simulink model "two_parallel_half_model_simscape"  (R2023b)
settings: Solver=ode1be  StartTime=0.0  StopTime=simlength  FixedStep=ts_sim  MaxStep=ts_sim
values from neighbouring files (symbols this model uses):
  fPWM_INV = 10e3    (= 10000)    [init_model.m]
  I_FS = Iout_ac_rms_nom * sqrt(2) * margin_factor    [init_model.m]
  ki_i_inv = 18    [init_model.m]
  ki_v_inv = 12.5    [init_model.m]
  kp_i_inv = 0.1    [init_model.m]
  kp_v_inv = 0.1    [init_model.m]
  LFu_ac = 125e-6*2    (= 0.00025)    [init_model.m]
  omega_grid = frequency_grid*2*pi    (= 314.159265359)    [init_model.m]
  RLFu_ac = 2e-3    (= 0.002)    [init_model.m]
  tc = ts_inv/200    (= 5e-07)    [init_model.m]
  ts_afe = ts_inv    (= 0.0001)    [init_model.m]
  ts_inv = tPWM_INV    (= 0.0001)    [init_model.m]
  ts_zvs = tPWM_ZVS*2    (= 0.0001)    [init_model.m]
  V_FS = Vout_dc_nom * margin_factor    (= 943)    [init_model.m]
  Vout_dc_nom = 820    [init_model.m]
undefined symbols (not defined in the file or in its folder): magnitude
libraries: fl_lib x43, nesl_utility x17
(part 1 of 2)
settings Model: SimulationMode=accelerator  Creator=LTNBDA  LastModifiedBy=dbagn
settings SolverCC: ZeroCrossControl=EnableAll  ZeroCrossAlgorithm=Adaptive  AlgebraicLoopSolver=TrustRegion  SolverResetMethod=Robust  AutoInsertRateTranBlk=on
settings DataIOCC: LimitDataPoints=on  MaxDataPoints=1  SaveFormat=Array  SignalLoggingSaveFormat=ModelDataLogs  SaveOutput=off  SignalLogging=off  DSMLogging=off  SaveTime=off  ReturnWorkspaceOutputs=off
settings OptimizationCC: ExpressionDepthLimit=2147483647  InitFltsAndDblsToZero=on  EfficientMapNaN2IntZero=off  LifeSpan=inf
settings DebuggingCC: SaveWithParameterizedLinksMsg=none  UnderspecifiedInitializationDetection=Classic  MergeDetectMultiDrivingBlocksExec=none  SignalResolutionControl=TryResolveAllWithWarning  SolverPrmCheckMsg=warning  MultiTaskDSMMsg=warning  MultiTaskCondExecSysMsg=none  MultiTaskRateTransMsg=warning  FcnCallInpInsideContextMsg=warning  StateNameClashWarn=warning  SFUnexpectedBacktrackingDiag=warning  SFNoUnconditionalDefaultTransitionDiag=warning  ArithmeticOperatorsInVariantConditions=warning
settings HardwareCC: ProdBitPerLong=64  ProdLargestAtomicFloat=None  ProdIntDivRoundTo=Undefined  ProdEndianess=Unspecified  ProdHWDeviceType=Generic->64-bit Embedded Processor (LP64)  TargetBitPerPointer=64  TargetBitPerSizeT=64  TargetBitPerPtrDiffT=64  TargetLongLongMode=on  TargetIntDivRoundTo=Zero  TargetEndianess=LittleEndian  TargetWordSize=64  TargetHWDeviceType=MATLAB Host  ProdEqTarget=off
settings ModelReferenceCC: EnableRefExpFcnMdlSchedulingChecks=on  PropagateSignalLabelsOutOfModel=off
settings SFSimCC: SimUseLocalCustomCode=off  CustomCodeUndefinedFunction=UseInterfaceOnly
settings RTWCC: RTWUseLocalCustomCode=off
settings CodeAppCC: MaxIdLength=128  StateflowObjectComments=on
settings GRTTargetCC: TargetLangStandard=C89/C90 (ANSI)  CombineOutputUpdateFcns=off  GRTInterface=on
settings ConfigComp: CovMetricSettings=dw  CovSaveCumulativeToWorkspaceVar=on  CovSaveSingleToWorkspaceVar=on  CovExternalEMLEnable=off
settings SimscapeCC: SimscapeNormalizeSystem=off

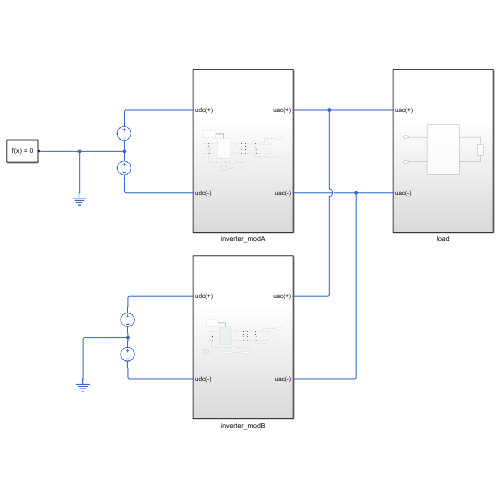
[thumbnail: Simulink's stored preview of the top-level diagram]
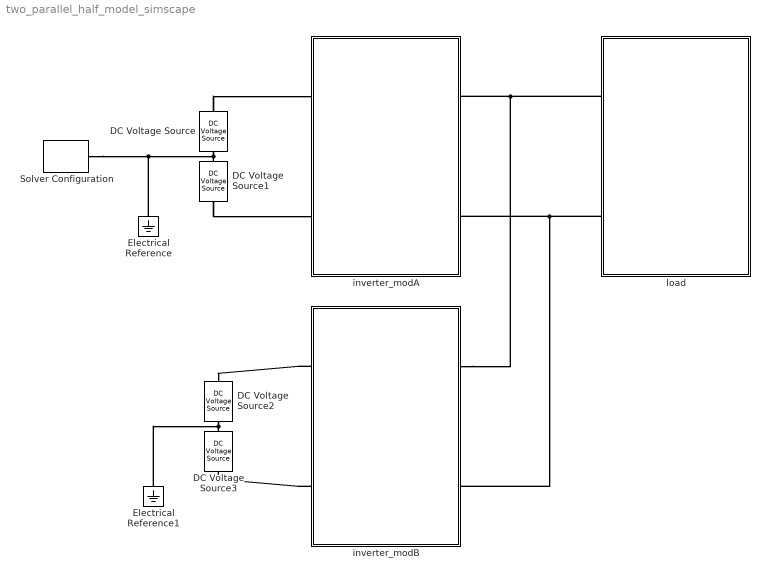
== system two_parallel_half_model_simscape ==
  DC Voltage Source{,1..3} (4 alike) : fl_lib/Electrical/Electrical Sources/DC Voltage Source  v0=Vout_dc_nom/2 V
  Electrical Reference : fl_lib/Electrical/Electrical Elements/Electrical Reference
  Electrical Reference1 : fl_lib/Electrical/Electrical Elements/Electrical Reference
  Solver Configuration : nesl_utility/Solver Configuration  PhysicalDomain=network_engine_domain  SubClassName=solver  LeftPortType=input  RightPortType=generic  Tones=[]  Harmonics=[]  SimulateNoise=off  Profile=off  UseLocalSampling=off  EnableSwitchedLinearOptims=on  FrequencyDomain=off  UseCCode=off  RelTol=0.001  AbsTol=0.001  MinStep=1e-09  ToWorkspace=off  RevertToSquareIcSolve=off  NumHomotopyIterations=100  PhasorMode=off  PhasorModeNumHarmonics=1  ConsistencySolver=NEWTON_FTOL  IndexReductionMethod=DerivativeReplacement  DoDC=on  ResidualTolerance=1e-09  ConsistencyTolSource=GLOBAL  ConsistencyAbsTol=0.001  ConsistencyRelTol=0.001  ConsistencyTolFactor=0.001  UseLocalSolver=on  LocalSolverChoice=NE_BACKWARD_EULER_ADVANCER  ResolveIndetEquations=on  FunctionEvalNumThread=1  LocalSolverSampleTime=ts_sim  DoFixedCost=on  MaxNonlinIter=3  MaxModeIter=2  ComputeImpulses=off  ImpulseIterations=2  LinearAlgebra=auto  LinearAlgebraNumThread=0  EquationFormulation=NE_TIME_EF  DelaysMemoryBudget=1024  AutomaticFiltering=on  FilteringTimeConstant=0.001  PartitionStorageMethod=AS_NEEDED  PartitionMemoryBudget=1024  PartitionMethod=ROBUST  MultibodyUseLocalSolver=off  MultibodyLocalSolverChoice=ODE1  MultibodyLocalSolverSampleTime=0.001
  inverter_modA : Subsystem
  inverter_modB : Subsystem
  load : Subsystem
  connections:
  DC Voltage Source/LConn1 -- inverter_modA/LConn1
  DC Voltage Source1/RConn1 -- inverter_modA/LConn2
  load/LConn1 -- inverter_modB/RConn1 -- inverter_modA/RConn1
  load/LConn2 -- inverter_modB/RConn2 -- inverter_modA/RConn2
  Solver Configuration/RConn1 -- Electrical Reference/LConn1 -- DC Voltage Source1/LConn1 -- DC Voltage Source/RConn1
  Electrical Reference1/LConn1 -- DC Voltage Source2/RConn1 -- DC Voltage Source3/LConn1
  inverter_modB/LConn2 -- DC Voltage Source3/RConn1
  inverter_modB/LConn1 -- DC Voltage Source2/LConn1

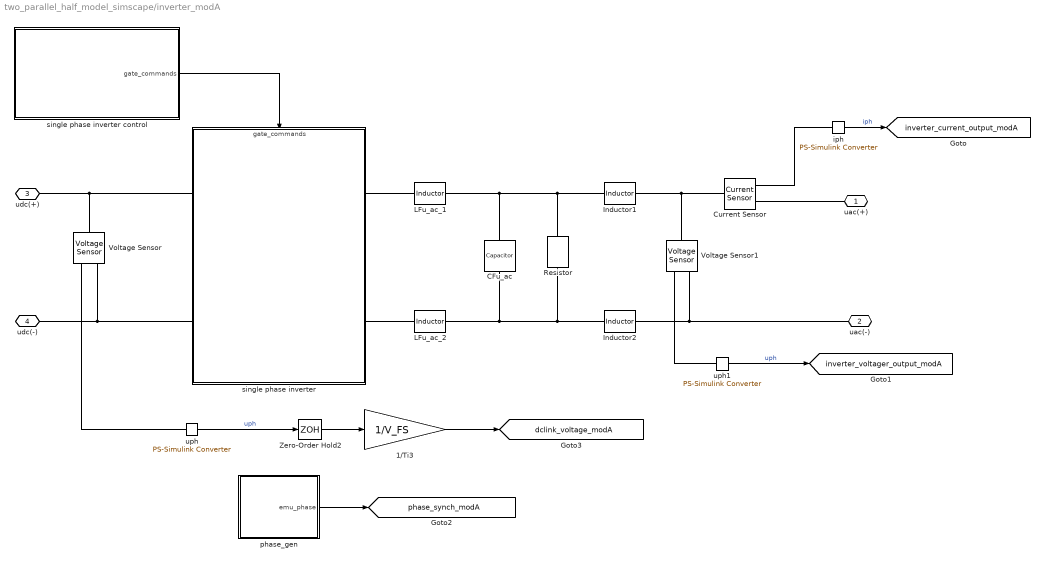
== system two_parallel_half_model_simscape/inverter_modA ==
  1/Ti3 : Gain  Gain=1/V_FS  SaturateOnIntegerOverflow=on  OutDataTypeStr=Inherit: Same as input  ParamDataTypeStr=Inherit: Same as input
  CFu_ac : fl_lib/Electrical/Electrical Elements/Capacitor  c=CFu_ac F  r=RCFu_ac Ohm  g=0 1/Ohm  i_specify=off  i_priority=None  i=0 A  i_nominal_specify=off  i_nominal_unit=A  i_nominal_value=1  v_specify=off  v_priority=None  v=0 V  v_nominal_specify=off  v_nominal_unit=V  v_nominal_value=1  vc_specify=off  vc_priority=High  vc=0 V  vc_nominal_specify=off  vc_nominal_unit=V  vc_nominal_value=1
  Current Sensor : fl_lib/Electrical/Electrical Sensors/Current Sensor
  Inductor1 : fl_lib/Electrical/Electrical Elements/Inductor  l=Lp H  r=0 Ohm  g=1e-9 1/Ohm  i_specify=off  i_priority=None  i=0 A  i_nominal_specify=off  i_nominal_unit=A  i_nominal_value=1  v_specify=off  v_priority=None  v=0 V  v_nominal_specify=off  v_nominal_unit=V  v_nominal_value=1  i_L_specify=off  i_L_priority=High  i_L=0 A  i_L_nominal_specify=off  i_L_nominal_unit=A  i_L_nominal_value=1
  Inductor2 : fl_lib/Electrical/Electrical Elements/Inductor  l=Lp H  r=0 Ohm  g=1e-9 1/Ohm  i_specify=off  i_priority=None  i=0 A  i_nominal_specify=off  i_nominal_unit=A  i_nominal_value=1  v_specify=off  v_priority=None  v=0 V  v_nominal_specify=off  v_nominal_unit=V  v_nominal_value=1  i_L_specify=off  i_L_priority=High  i_L=0 A  i_L_nominal_specify=off  i_L_nominal_unit=A  i_L_nominal_value=1
  LFu_ac_1 : fl_lib/Electrical/Electrical Elements/Inductor  l=LFu_ac/2 H  r=RLFu_ac/2 Ohm  g=0 1/Ohm  i_specify=off  i_priority=None  i=0 A  i_nominal_specify=off  i_nominal_unit=A  i_nominal_value=1  v_specify=off  v_priority=None  v=0 V  v_nominal_specify=off  v_nominal_unit=V  v_nominal_value=1  i_L_specify=off  i_L_priority=High  i_L=0 A  i_L_nominal_specify=off  i_L_nominal_unit=A  i_L_nominal_value=1
  LFu_ac_2 : fl_lib/Electrical/Electrical Elements/Inductor  l=LFu_ac/2 H  r=RLFu_ac/2 Ohm  g=0 1/Ohm  i_specify=off  i_priority=None  i=0 A  i_nominal_specify=off  i_nominal_unit=A  i_nominal_value=1  v_specify=off  v_priority=None  v=0 V  v_nominal_specify=off  v_nominal_unit=V  v_nominal_value=1  i_L_specify=off  i_L_priority=High  i_L=0 A  i_L_nominal_specify=off  i_L_nominal_unit=A  i_L_nominal_value=1
  Resistor : fl_lib/Electrical/Electrical Elements/Resistor  R=10e3 Ohm  i_specify=off  i_priority=None  i=0 A  i_nominal_specify=off  i_nominal_unit=A  i_nominal_value=1  v_specify=off  v_priority=None  v=0 V  v_nominal_specify=off  v_nominal_unit=V  v_nominal_value=1
  Voltage Sensor : fl_lib/Electrical/Electrical Sensors/Voltage Sensor
  Voltage Sensor1 : fl_lib/Electrical/Electrical Sensors/Voltage Sensor
  Zero-Order Hold2 : ZeroOrderHold  SampleTime=ts_zvs
  iph : nesl_utility/PS-Simulink Converter  PhysicalDomain=network_engine_domain  SubClassName=ps_output  LeftPortType=input  RightPortType=output  PseudoPeriodic=off  Frequencies=[]  VectorFormat=1-D array  Unit=A  AffineConversion=off
  phase_gen : Subsystem
  single phase inverter : Subsystem
      settings: PortSchema="{\"entries\":[{\"content\":{\"sides\":[{\"content\":{\"connectorIds\":[\"LConn1\",\"LConn2\"]},\"type\":\"ConnectorPlacement.EquallySpacedRectSide\",\"uuid\":\"4fcf4fea-d38f-431b-8a91-be3ce9782faf\"},{\"content\":{\"connectorIds\":[\"RConn1\",\"RConn2\"],\"side\":\"RIGHT\"},\"type\":\"ConnectorPlacement.EquallySpacedRectSide\",\"uuid\":\"0aa56277-92e9-4e3b-84c7-43398254a4d8\"},{\"content\":{\"connectorIds\":[\"In1\"],\"side\":\"TOP\"},\"type\":\"ConnectorPlacement.EquallySpacedRectSide\",\"uuid\":\"5cd150dc-bcaf-4cd7-b2a8-3db203726730\"}]},\"type\":\"ConnectorPlacement.EquallySpacedConnector\",\"uuid\":\"bf8194c4-c327-4d40-bea4-f1e7617f80b4\"}],\"packageUris\":[\"http://schema.mathworks.com/mf0/Connector/R2020b\"],\"version\":\"1.0\"}"
  single phase inverter control : Subsystem
  uph : nesl_utility/PS-Simulink Converter  PhysicalDomain=network_engine_domain  SubClassName=ps_output  LeftPortType=input  RightPortType=output  PseudoPeriodic=off  Frequencies=[]  VectorFormat=1-D array  Unit=V  AffineConversion=off
  uph1 : nesl_utility/PS-Simulink Converter  PhysicalDomain=network_engine_domain  SubClassName=ps_output  LeftPortType=input  RightPortType=output  PseudoPeriodic=off  Frequencies=[]  VectorFormat=1-D array  Unit=V  AffineConversion=off
  uac(+) : PMIOPort  Side=Right
  uac(-) : PMIOPort  Port=2  Side=Right
  udc(+) : PMIOPort  Port=3  Side=Left
  udc(-) : PMIOPort  Port=4  Side=Left
  tag scope: dclink_voltage_modA=global, inverter_current_output_modA=global, inverter_voltager_output_modA=global, phase_synch_modA=global
  wires:
  Zero-Order Hold2/1 -> 1/Ti3/1
  1/Ti3/1 -> [dclink_voltage_modA]
  single phase inverter control/1(gate_commands) -> single phase inverter/1(gate_commands)
  uph/1 -> Zero-Order Hold2/1  "uph"
  iph/1 -> [inverter_current_output_modA]  "iph"
  uph1/1 -> [inverter_voltager_output_modA]  "uph"
  phase_gen/1(emu_phase) -> [phase_synch_modA]
  connections:
  single phase inverter/RConn2 -- Voltage Sensor/RConn2 -- udc(-)/RConn1
  single phase inverter/RConn1 -- Voltage Sensor/LConn1 -- udc(+)/RConn1
  LFu_ac_1/LConn1 -- single phase inverter/LConn1
  Inductor1/RConn1 -- Voltage Sensor1/LConn1 -- Current Sensor/LConn1
  single phase inverter/LConn2 -- LFu_ac_2/RConn1
  LFu_ac_2/LConn1 -- Inductor2/LConn1 -- Resistor/RConn1 -- CFu_ac/RConn1
  Voltage Sensor/RConn1 -- uph/LConn1
  Voltage Sensor1/RConn1 -- uph1/LConn1
  Current Sensor/RConn1 -- iph/LConn1
  Voltage Sensor1/RConn2 -- Inductor2/RConn1 -- uac(-)/RConn1
  CFu_ac/LConn1 -- Inductor1/LConn1 -- Resistor/LConn1 -- LFu_ac_1/RConn1
  Current Sensor/RConn2 -- uac(+)/RConn1

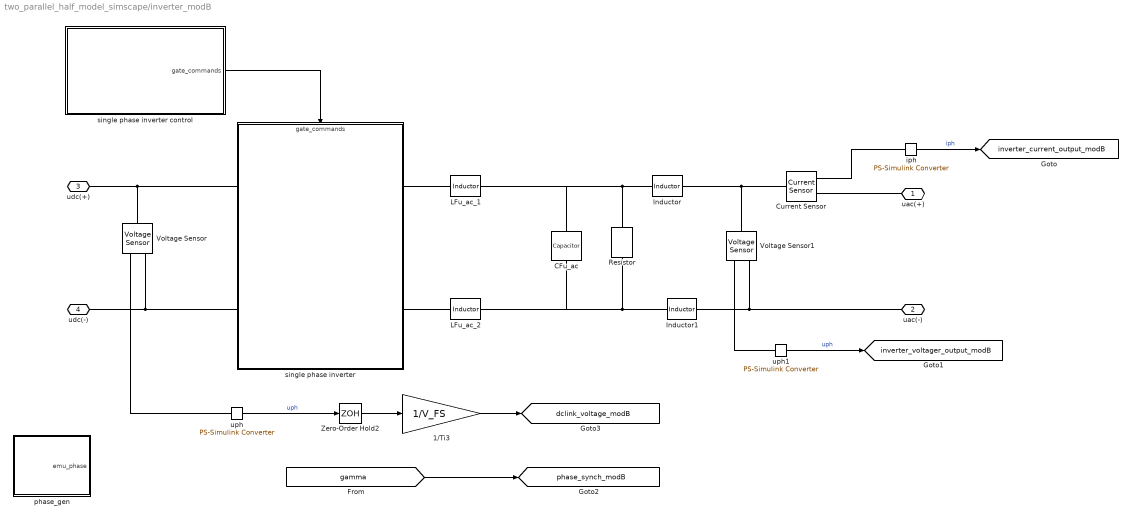
== system two_parallel_half_model_simscape/inverter_modB ==
  1/Ti3 : Gain  Gain=1/V_FS  SaturateOnIntegerOverflow=on  OutDataTypeStr=Inherit: Same as input  ParamDataTypeStr=Inherit: Same as input
  CFu_ac : fl_lib/Electrical/Electrical Elements/Capacitor  c=CFu_ac F  r=RCFu_ac Ohm  g=0 1/Ohm  i_specify=off  i_priority=None  i=0 A  i_nominal_specify=off  i_nominal_unit=A  i_nominal_value=1  v_specify=off  v_priority=None  v=0 V  v_nominal_specify=off  v_nominal_unit=V  v_nominal_value=1  vc_specify=off  vc_priority=High  vc=0 V  vc_nominal_specify=off  vc_nominal_unit=V  vc_nominal_value=1
  Current Sensor : fl_lib/Electrical/Electrical Sensors/Current Sensor
  Inductor : fl_lib/Electrical/Electrical Elements/Inductor  l=Lp H  r=0 Ohm  g=1e-9 1/Ohm  i_specify=off  i_priority=None  i=0 A  i_nominal_specify=off  i_nominal_unit=A  i_nominal_value=1  v_specify=off  v_priority=None  v=0 V  v_nominal_specify=off  v_nominal_unit=V  v_nominal_value=1  i_L_specify=off  i_L_priority=High  i_L=0 A  i_L_nominal_specify=off  i_L_nominal_unit=A  i_L_nominal_value=1
  Inductor1 : fl_lib/Electrical/Electrical Elements/Inductor  l=Lp H  r=0 Ohm  g=1e-9 1/Ohm  i_specify=off  i_priority=None  i=0 A  i_nominal_specify=off  i_nominal_unit=A  i_nominal_value=1  v_specify=off  v_priority=None  v=0 V  v_nominal_specify=off  v_nominal_unit=V  v_nominal_value=1  i_L_specify=off  i_L_priority=High  i_L=0 A  i_L_nominal_specify=off  i_L_nominal_unit=A  i_L_nominal_value=1
  LFu_ac_1 : fl_lib/Electrical/Electrical Elements/Inductor  l=LFu_ac/2 H  r=RLFu_ac/2 Ohm  g=0 1/Ohm  i_specify=off  i_priority=None  i=0 A  i_nominal_specify=off  i_nominal_unit=A  i_nominal_value=1  v_specify=off  v_priority=None  v=0 V  v_nominal_specify=off  v_nominal_unit=V  v_nominal_value=1  i_L_specify=off  i_L_priority=High  i_L=0 A  i_L_nominal_specify=off  i_L_nominal_unit=A  i_L_nominal_value=1
  LFu_ac_2 : fl_lib/Electrical/Electrical Elements/Inductor  l=LFu_ac/2 H  r=RLFu_ac/2 Ohm  g=0 1/Ohm  i_specify=off  i_priority=None  i=0 A  i_nominal_specify=off  i_nominal_unit=A  i_nominal_value=1  v_specify=off  v_priority=None  v=0 V  v_nominal_specify=off  v_nominal_unit=V  v_nominal_value=1  i_L_specify=off  i_L_priority=High  i_L=0 A  i_L_nominal_specify=off  i_L_nominal_unit=A  i_L_nominal_value=1
  Resistor : fl_lib/Electrical/Electrical Elements/Resistor  R=10e3 Ohm  i_specify=off  i_priority=None  i=0 A  i_nominal_specify=off  i_nominal_unit=A  i_nominal_value=1  v_specify=off  v_priority=None  v=0 V  v_nominal_specify=off  v_nominal_unit=V  v_nominal_value=1
  Voltage Sensor : fl_lib/Electrical/Electrical Sensors/Voltage Sensor
  Voltage Sensor1 : fl_lib/Electrical/Electrical Sensors/Voltage Sensor
  Zero-Order Hold2 : ZeroOrderHold  SampleTime=ts_zvs
  iph : nesl_utility/PS-Simulink Converter  PhysicalDomain=network_engine_domain  SubClassName=ps_output  LeftPortType=input  RightPortType=output  PseudoPeriodic=off  Frequencies=[]  VectorFormat=1-D array  Unit=A  AffineConversion=off
  phase_gen : Subsystem
  single phase inverter : Subsystem
      settings: PortSchema="{\"entries\":[{\"content\":{\"sides\":[{\"content\":{\"connectorIds\":[\"LConn1\",\"LConn2\"]},\"type\":\"ConnectorPlacement.EquallySpacedRectSide\",\"uuid\":\"4fcf4fea-d38f-431b-8a91-be3ce9782faf\"},{\"content\":{\"connectorIds\":[\"RConn1\",\"RConn2\"],\"side\":\"RIGHT\"},\"type\":\"ConnectorPlacement.EquallySpacedRectSide\",\"uuid\":\"0aa56277-92e9-4e3b-84c7-43398254a4d8\"},{\"content\":{\"connectorIds\":[\"In1\"],\"side\":\"TOP\"},\"type\":\"ConnectorPlacement.EquallySpacedRectSide\",\"uuid\":\"5cd150dc-bcaf-4cd7-b2a8-3db203726730\"}]},\"type\":\"ConnectorPlacement.EquallySpacedConnector\",\"uuid\":\"bf8194c4-c327-4d40-bea4-f1e7617f80b4\"}],\"packageUris\":[\"http://schema.mathworks.com/mf0/Connector/R2020b\"],\"version\":\"1.0\"}"
  single phase inverter control : Subsystem
  uph : nesl_utility/PS-Simulink Converter  PhysicalDomain=network_engine_domain  SubClassName=ps_output  LeftPortType=input  RightPortType=output  PseudoPeriodic=off  Frequencies=[]  VectorFormat=1-D array  Unit=V  AffineConversion=off
  uph1 : nesl_utility/PS-Simulink Converter  PhysicalDomain=network_engine_domain  SubClassName=ps_output  LeftPortType=input  RightPortType=output  PseudoPeriodic=off  Frequencies=[]  VectorFormat=1-D array  Unit=V  AffineConversion=off
  uac(+) : PMIOPort  Side=Right
  uac(-) : PMIOPort  Port=2  Side=Right
  udc(+) : PMIOPort  Port=3  Side=Left
  udc(-) : PMIOPort  Port=4  Side=Left
  tag scope: dclink_voltage_modB=global, inverter_current_output_modB=global, inverter_voltager_output_modB=global, phase_synch_modB=global
  wires:
  uph1/1 -> [inverter_voltager_output_modB]  "uph"
  iph/1 -> [inverter_current_output_modB]  "iph"
  uph/1 -> Zero-Order Hold2/1  "uph"
  single phase inverter control/1(gate_commands) -> single phase inverter/1(gate_commands)
  1/Ti3/1 -> [dclink_voltage_modB]
  Zero-Order Hold2/1 -> 1/Ti3/1
  [gamma] -> [phase_synch_modB]
  connections:
  Current Sensor/RConn1 -- iph/LConn1
  Voltage Sensor1/RConn1 -- uph1/LConn1
  Voltage Sensor/RConn1 -- uph/LConn1
  Voltage Sensor1/RConn2 -- Inductor1/RConn1 -- uac(-)/RConn1
  single phase inverter/LConn2 -- LFu_ac_2/RConn1
  Inductor/RConn1 -- Voltage Sensor1/LConn1 -- Current Sensor/LConn1
  LFu_ac_1/LConn1 -- single phase inverter/LConn1
  Voltage Sensor/LConn1 -- single phase inverter/RConn1 -- udc(+)/RConn1
  Voltage Sensor/RConn2 -- udc(-)/RConn1 -- single phase inverter/RConn2
  Resistor/LConn1 -- CFu_ac/LConn1 -- LFu_ac_1/RConn1 -- Inductor/LConn1
  Resistor/RConn1 -- Inductor1/LConn1 -- LFu_ac_2/LConn1 -- CFu_ac/RConn1
  Current Sensor/RConn2 -- uac(+)/RConn1

== system two_parallel_half_model_simscape/load ==
  RL-load : fl_lib/Electrical/Electrical Elements/Inductor  l=Lload H  r=Rload Ohm  g=0 1/Ohm  i_specify=off  i_priority=None  i=0 A  i_nominal_specify=off  i_nominal_unit=A  i_nominal_value=1  v_specify=off  v_priority=None  v=0 V  v_nominal_specify=off  v_nominal_unit=V  v_nominal_value=1  i_L_specify=off  i_L_priority=High  i_L=0 A  i_L_nominal_specify=off  i_L_nominal_unit=A  i_L_nominal_value=1
  single_phase_ui_measure : Subsystem
  uac(+) : PMIOPort  Side=Left
  uac(-) : PMIOPort  Port=2  Side=Left
  connections:
  single_phase_ui_measure/LConn1 -- uac(+)/RConn1
  uac(-)/RConn1 -- single_phase_ui_measure/LConn2
  single_phase_ui_measure/RConn1 -- RL-load/LConn1
  RL-load/RConn1 -- single_phase_ui_measure/RConn2

== system two_parallel_half_model_simscape/inverter_modA/phase_gen ==
  Constant4 : Constant  Value=omega_grid
  Integrator : Integrator
  bounder1 : MATLAB Function  TreatAsAtomicUnit=on  SystemSampleTime=ts_afe
  emu_phase : Outport  VectorParamsAs1DForOutWhenUnconnected=off
  tag scope: gamma=global
  wires:
  bounder1/1(y) -> [gamma], emu_phase/1  "emu_phase"
  Constant4/1 -> Integrator/1
  Integrator/1 -> bounder1/1(u)

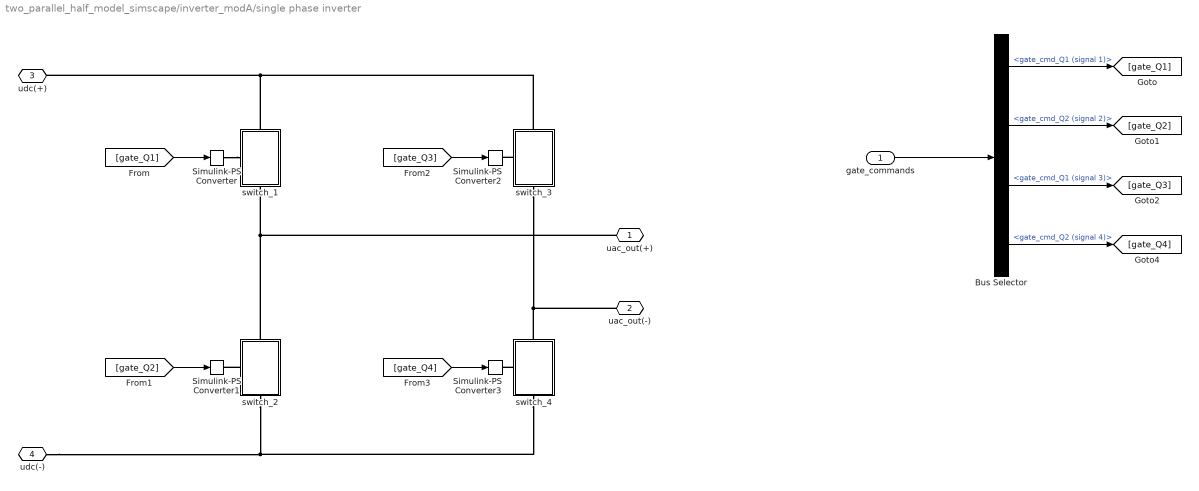
== system two_parallel_half_model_simscape/inverter_modA/single phase inverter ==
  gate_commands : Inport
  Bus Selector : BusSelector  OutputSignals=gate_cmd_Q1 (signal 1),gate_cmd_Q2 (signal 2),gate_cmd_Q1 (signal 3),gate_cmd_Q2 (signal 4)
  Simulink-PS Converter{,1..3} (4 alike) : nesl_utility/Simulink-PS Converter  PhysicalDomain=network_engine_domain  SubClassName=ps_input  LeftPortType=input  RightPortType=output  PseudoPeriodic=off  Frequencies=[]  NoiseDistribution=none  NoiseParameters=[]  Unit=1  AffineConversion=on  FilteringAndDerivatives=provide  SimscapeFilterOrder=1  InputFilterTimeConstant=0.001  UdotUserProvided=0
  switch_1 : Subsystem
      settings: PortSchema="{\"entries\":[{\"content\":{\"sides\":[{\"content\":{\"connectorIds\":[\"LConn1\"]},\"type\":\"ConnectorPlacement.EquallySpacedRectSide\",\"uuid\":\"9277da8d-d460-43e6-8478-dd662f15d226\"},{\"content\":{\"connectorIds\":[],\"side\":\"RIGHT\"},\"type\":\"ConnectorPlacement.EquallySpacedRectSide\",\"uuid\":\"a7ece396-f1d9-4f4f-a05b-db1fc65d6e1d\"},{\"content\":{\"connectorIds\":[\"LConn2\"],\"side\":\"TOP\"},\"type\":\"ConnectorPlacement.EquallySpacedRectSide\",\"uuid\":\"fdd70777-e9cf-4317-afb6-cae87f75d5b0\"},{\"content\":{\"connectorIds\":[\"RConn1\"],\"side\":\"BOTTOM\"},\"type\":\"ConnectorPlacement.EquallySpacedRectSide\",\"uuid\":\"2353ed68-b1a1-4775-9ca9-31e268d5443b\"}]},\"type\":\"ConnectorPlacement.EquallySpacedConnector\",\"uuid\":\"d5479f4c-4e65-4791-adcb-73df11f88590\"}],\"packageUris\":[\"http://schema.mathworks.com/mf0/Connector/R2020b\"],\"version\":\"1.0\"}"
  switch_2 : Subsystem
      settings: PortSchema="{\"entries\":[{\"content\":{\"sides\":[{\"content\":{\"connectorIds\":[\"LConn1\"]},\"type\":\"ConnectorPlacement.EquallySpacedRectSide\",\"uuid\":\"9277da8d-d460-43e6-8478-dd662f15d226\"},{\"content\":{\"connectorIds\":[],\"side\":\"RIGHT\"},\"type\":\"ConnectorPlacement.EquallySpacedRectSide\",\"uuid\":\"a7ece396-f1d9-4f4f-a05b-db1fc65d6e1d\"},{\"content\":{\"connectorIds\":[\"LConn2\"],\"side\":\"TOP\"},\"type\":\"ConnectorPlacement.EquallySpacedRectSide\",\"uuid\":\"fdd70777-e9cf-4317-afb6-cae87f75d5b0\"},{\"content\":{\"connectorIds\":[\"RConn1\"],\"side\":\"BOTTOM\"},\"type\":\"ConnectorPlacement.EquallySpacedRectSide\",\"uuid\":\"2353ed68-b1a1-4775-9ca9-31e268d5443b\"}]},\"type\":\"ConnectorPlacement.EquallySpacedConnector\",\"uuid\":\"d5479f4c-4e65-4791-adcb-73df11f88590\"}],\"packageUris\":[\"http://schema.mathworks.com/mf0/Connector/R2020b\"],\"version\":\"1.0\"}"
  switch_3 : Subsystem
      settings: PortSchema="{\"entries\":[{\"content\":{\"sides\":[{\"content\":{\"connectorIds\":[\"LConn1\"]},\"type\":\"ConnectorPlacement.EquallySpacedRectSide\",\"uuid\":\"9277da8d-d460-43e6-8478-dd662f15d226\"},{\"content\":{\"connectorIds\":[],\"side\":\"RIGHT\"},\"type\":\"ConnectorPlacement.EquallySpacedRectSide\",\"uuid\":\"a7ece396-f1d9-4f4f-a05b-db1fc65d6e1d\"},{\"content\":{\"connectorIds\":[\"LConn2\"],\"side\":\"TOP\"},\"type\":\"ConnectorPlacement.EquallySpacedRectSide\",\"uuid\":\"fdd70777-e9cf-4317-afb6-cae87f75d5b0\"},{\"content\":{\"connectorIds\":[\"RConn1\"],\"side\":\"BOTTOM\"},\"type\":\"ConnectorPlacement.EquallySpacedRectSide\",\"uuid\":\"2353ed68-b1a1-4775-9ca9-31e268d5443b\"}]},\"type\":\"ConnectorPlacement.EquallySpacedConnector\",\"uuid\":\"d5479f4c-4e65-4791-adcb-73df11f88590\"}],\"packageUris\":[\"http://schema.mathworks.com/mf0/Connector/R2020b\"],\"version\":\"1.0\"}"
  switch_4 : Subsystem
      settings: PortSchema="{\"entries\":[{\"content\":{\"sides\":[{\"content\":{\"connectorIds\":[\"LConn1\"]},\"type\":\"ConnectorPlacement.EquallySpacedRectSide\",\"uuid\":\"9277da8d-d460-43e6-8478-dd662f15d226\"},{\"content\":{\"connectorIds\":[],\"side\":\"RIGHT\"},\"type\":\"ConnectorPlacement.EquallySpacedRectSide\",\"uuid\":\"a7ece396-f1d9-4f4f-a05b-db1fc65d6e1d\"},{\"content\":{\"connectorIds\":[\"LConn2\"],\"side\":\"TOP\"},\"type\":\"ConnectorPlacement.EquallySpacedRectSide\",\"uuid\":\"fdd70777-e9cf-4317-afb6-cae87f75d5b0\"},{\"content\":{\"connectorIds\":[\"RConn1\"],\"side\":\"BOTTOM\"},\"type\":\"ConnectorPlacement.EquallySpacedRectSide\",\"uuid\":\"2353ed68-b1a1-4775-9ca9-31e268d5443b\"}]},\"type\":\"ConnectorPlacement.EquallySpacedConnector\",\"uuid\":\"d5479f4c-4e65-4791-adcb-73df11f88590\"}],\"packageUris\":[\"http://schema.mathworks.com/mf0/Connector/R2020b\"],\"version\":\"1.0\"}"
  uac_out(+) : PMIOPort  Side=Left
  uac_out(-) : PMIOPort  Port=2  Side=Left
  udc(+) : PMIOPort  Port=3  Side=Right
  udc(-) : PMIOPort  Port=4  Side=Right
  wires:
  [gate_Q1] -> Simulink-PS Converter/1
  [gate_Q2] -> Simulink-PS Converter1/1
  [gate_Q3] -> Simulink-PS Converter2/1
  [gate_Q4] -> Simulink-PS Converter3/1
  gate_commands/1 -> Bus Selector/1
  Bus Selector/1 -> [gate_Q1]  "<gate_cmd_Q1 (signal 1)>"
  Bus Selector/2 -> [gate_Q2]  "<gate_cmd_Q2 (signal 2)>"
  Bus Selector/3 -> [gate_Q3]  "<gate_cmd_Q1 (signal 3)>"
  Bus Selector/4 -> [gate_Q4]  "<gate_cmd_Q2 (signal 4)>"
  connections:
  switch_3/LConn2 -- switch_1/LConn2 -- udc(+)/RConn1
  udc(-)/RConn1 -- switch_4/RConn1 -- switch_2/RConn1
  Simulink-PS Converter/RConn1 -- switch_1/LConn1
  switch_2/LConn1 -- Simulink-PS Converter1/RConn1
  switch_3/LConn1 -- Simulink-PS Converter2/RConn1
  switch_4/LConn1 -- Simulink-PS Converter3/RConn1
  uac_out(+)/RConn1 -- switch_2/LConn2 -- switch_1/RConn1
  uac_out(-)/RConn1 -- switch_4/LConn2 -- switch_3/RConn1

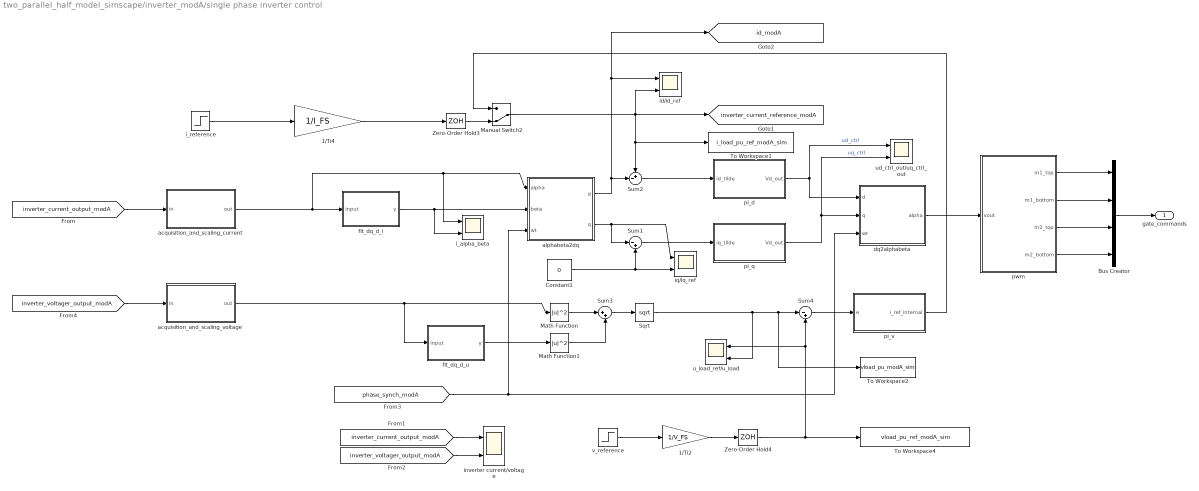
== system two_parallel_half_model_simscape/inverter_modA/single phase inverter control ==
  1/Ti2 : Gain  Gain=1/V_FS  SaturateOnIntegerOverflow=on  OutDataTypeStr=Inherit: Same as input  ParamDataTypeStr=Inherit: Same as input
  1/Ti4 : Gain  Gain=1/I_FS  SaturateOnIntegerOverflow=on  OutDataTypeStr=Inherit: Same as input  ParamDataTypeStr=Inherit: Same as input
  Bus Creator : BusCreator  Inputs=4
  Constant1 : Constant  Value=0
  Manual Switch2 : ManualSwitch  CurrentSetting=0
  Math Function : Math  Operator=magnitude^2
  Math Function1 : Math  Operator=magnitude^2
  Sqrt : Sqrt
  Sum1 : Sum  Inputs=|-+
  Sum2 : Sum  Inputs=+-|
  Sum3 : Sum  Inputs=|++
  Sum4 : Sum  Inputs=|-+
  To Workspace1 : ToWorkspace  VariableName=i_load_pu_ref_modA_sim  SampleTime=ts_inv
      settings: MaxDataPoints=Ns_inv
  To Workspace2 : ToWorkspace  VariableName=vload_pu_modA_sim  SampleTime=ts_inv
      settings: MaxDataPoints=Ns_inv
  To Workspace4 : ToWorkspace  VariableName=vload_pu_ref_modA_sim  SampleTime=ts_inv
      settings: MaxDataPoints=Ns_inv
  Zero-Order Hold3 : ZeroOrderHold  SampleTime=ts_inv
  Zero-Order Hold4 : ZeroOrderHold  SampleTime=ts_inv
  acquisition_and_scaling_current : Subsystem
  acquisition_and_scaling_voltage : Subsystem
  alphabeta2dq : Subsystem
  dq2alphabeta : Subsystem
  flt_dq_d_i : MATLAB Function  TreatAsAtomicUnit=on  SystemSampleTime=ts_inv
  flt_dq_d_u : MATLAB Function  TreatAsAtomicUnit=on  SystemSampleTime=ts_inv
  i_alpha_beta : Scope  NumInputPorts=2
  i_reference : Step  Time=0.1  After=55*sqrt(2)  SampleTime=0
  id/id_ref : Scope  NumInputPorts=2
  inverter current/voltage : Scope  NumInputPorts=2
  iq/iq_ref : Scope  NumInputPorts=2
  pi_d : Subsystem
  pi_q : Subsystem
  pi_v : Subsystem
  pwm : Subsystem
  u_load_ref/u_load : Scope  NumInputPorts=2
  ud_ctrl_out/uq_ctrl_out : Scope  NumInputPorts=2
  v_reference : Step  Time=0.1  After=500*sqrt(2)  SampleTime=0
  gate_commands : Outport
  tag scope: id_modA=global, inverter_current_reference_modA=global
  wires:
  dq2alphabeta/1(alpha) -> pwm/1(vout)
  i_reference/1 -> 1/Ti4/1
  1/Ti4/1 -> Zero-Order Hold3/1
  flt_dq_d_i/1(y) -> i_alpha_beta/2, alphabeta2dq/2(beta)
  [phase_synch_modA] -> alphabeta2dq/3(wt), dq2alphabeta/3(wt)
  alphabeta2dq/2("q ") -> Sum1/1, iq/iq_ref/1
  alphabeta2dq/1("d ") -> [id_modA], id/id_ref/1, Sum2/2
  Zero-Order Hold3/1 -> Manual Switch2/2
  Manual Switch2/1 -> id/id_ref/2, [inverter_current_reference_modA], Sum2/1, To Workspace1/1
  Constant1/1 -> iq/iq_ref/2, Sum1/2
  Sum2/1 -> pi_d/1(id_tilde)
  Sum1/1 -> pi_q/1(iq_tilde)
  pi_d/1(Vd_out) -> ud_ctrl_out/uq_ctrl_out/1, dq2alphabeta/1(d)  "ud_ctrl"
  pi_q/1(Vd_out) -> dq2alphabeta/2(q), ud_ctrl_out/uq_ctrl_out/2  "uq_ctrl"
  flt_dq_d_u/1(y) -> Math Function1/1
  Math Function/1 -> Sum3/1
  Math Function1/1 -> Sum3/2
  Sum3/1 -> Sqrt/1
  1/Ti2/1 -> Zero-Order Hold4/1
  v_reference/1 -> 1/Ti2/1
  Sqrt/1 -> u_load_ref/u_load/2, To Workspace2/1, Sum4/1
  Zero-Order Hold4/1 -> Sum4/2, u_load_ref/u_load/1, To Workspace4/1
  Sum4/1 -> pi_v/1(e)
  pi_v/1(i_ref_internal) -> Manual Switch2/1
  pwm/3(m2_top) -> Bus Creator/3
  Bus Creator/1 -> gate_commands/1
  pwm/1(m1_top) -> Bus Creator/1
  pwm/2(m1_bottom) -> Bus Creator/2
  pwm/4(m2_bottom) -> Bus Creator/4
  acquisition_and_scaling_current/1(out) -> flt_dq_d_i/1(input), i_alpha_beta/1, alphabeta2dq/1(alpha)
  [inverter_current_output_modA] -> acquisition_and_scaling_current/1(in)
  acquisition_and_scaling_voltage/1(out) -> flt_dq_d_u/1(input), Math Function/1
  [inverter_voltager_output_modA] -> acquisition_and_scaling_voltage/1(in)
  [inverter_current_output_modA] -> inverter current/voltage/1
  [inverter_voltager_output_modA] -> inverter current/voltage/2

== system two_parallel_half_model_simscape/inverter_modB/phase_gen ==
  Constant4 : Constant  Value=omega_grid
  Integrator : Integrator
  bounder1 : MATLAB Function  TreatAsAtomicUnit=on  SystemSampleTime=ts_afe
  emu_phase : Outport  VectorParamsAs1DForOutWhenUnconnected=off
  wires:
  bounder1/1(y) -> emu_phase/1  "emu_phase"
  Constant4/1 -> Integrator/1
  Integrator/1 -> bounder1/1(u)

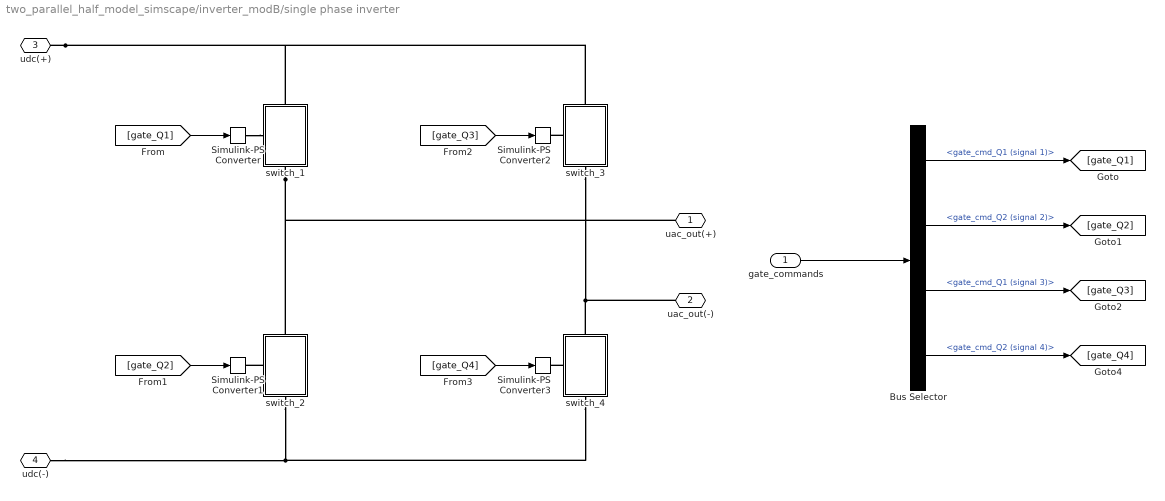
== system two_parallel_half_model_simscape/inverter_modB/single phase inverter ==
  gate_commands : Inport
  Bus Selector : BusSelector  OutputSignals=gate_cmd_Q1 (signal 1),gate_cmd_Q2 (signal 2),gate_cmd_Q1 (signal 3),gate_cmd_Q2 (signal 4)
  Simulink-PS Converter{,1..3} (4 alike) : nesl_utility/Simulink-PS Converter  PhysicalDomain=network_engine_domain  SubClassName=ps_input  LeftPortType=input  RightPortType=output  PseudoPeriodic=off  Frequencies=[]  NoiseDistribution=none  NoiseParameters=[]  Unit=1  AffineConversion=on  FilteringAndDerivatives=provide  SimscapeFilterOrder=1  InputFilterTimeConstant=0.001  UdotUserProvided=0
  switch_1 : Subsystem
      settings: PortSchema="{\"entries\":[{\"content\":{\"sides\":[{\"content\":{\"connectorIds\":[\"LConn1\"]},\"type\":\"ConnectorPlacement.EquallySpacedRectSide\",\"uuid\":\"9277da8d-d460-43e6-8478-dd662f15d226\"},{\"content\":{\"connectorIds\":[],\"side\":\"RIGHT\"},\"type\":\"ConnectorPlacement.EquallySpacedRectSide\",\"uuid\":\"a7ece396-f1d9-4f4f-a05b-db1fc65d6e1d\"},{\"content\":{\"connectorIds\":[\"LConn2\"],\"side\":\"TOP\"},\"type\":\"ConnectorPlacement.EquallySpacedRectSide\",\"uuid\":\"fdd70777-e9cf-4317-afb6-cae87f75d5b0\"},{\"content\":{\"connectorIds\":[\"RConn1\"],\"side\":\"BOTTOM\"},\"type\":\"ConnectorPlacement.EquallySpacedRectSide\",\"uuid\":\"2353ed68-b1a1-4775-9ca9-31e268d5443b\"}]},\"type\":\"ConnectorPlacement.EquallySpacedConnector\",\"uuid\":\"d5479f4c-4e65-4791-adcb-73df11f88590\"}],\"packageUris\":[\"http://schema.mathworks.com/mf0/Connector/R2020b\"],\"version\":\"1.0\"}"
  switch_2 : Subsystem
      settings: PortSchema="{\"entries\":[{\"content\":{\"sides\":[{\"content\":{\"connectorIds\":[\"LConn1\"]},\"type\":\"ConnectorPlacement.EquallySpacedRectSide\",\"uuid\":\"9277da8d-d460-43e6-8478-dd662f15d226\"},{\"content\":{\"connectorIds\":[],\"side\":\"RIGHT\"},\"type\":\"ConnectorPlacement.EquallySpacedRectSide\",\"uuid\":\"a7ece396-f1d9-4f4f-a05b-db1fc65d6e1d\"},{\"content\":{\"connectorIds\":[\"LConn2\"],\"side\":\"TOP\"},\"type\":\"ConnectorPlacement.EquallySpacedRectSide\",\"uuid\":\"fdd70777-e9cf-4317-afb6-cae87f75d5b0\"},{\"content\":{\"connectorIds\":[\"RConn1\"],\"side\":\"BOTTOM\"},\"type\":\"ConnectorPlacement.EquallySpacedRectSide\",\"uuid\":\"2353ed68-b1a1-4775-9ca9-31e268d5443b\"}]},\"type\":\"ConnectorPlacement.EquallySpacedConnector\",\"uuid\":\"d5479f4c-4e65-4791-adcb-73df11f88590\"}],\"packageUris\":[\"http://schema.mathworks.com/mf0/Connector/R2020b\"],\"version\":\"1.0\"}"
  switch_3 : Subsystem
      settings: PortSchema="{\"entries\":[{\"content\":{\"sides\":[{\"content\":{\"connectorIds\":[\"LConn1\"]},\"type\":\"ConnectorPlacement.EquallySpacedRectSide\",\"uuid\":\"9277da8d-d460-43e6-8478-dd662f15d226\"},{\"content\":{\"connectorIds\":[],\"side\":\"RIGHT\"},\"type\":\"ConnectorPlacement.EquallySpacedRectSide\",\"uuid\":\"a7ece396-f1d9-4f4f-a05b-db1fc65d6e1d\"},{\"content\":{\"connectorIds\":[\"LConn2\"],\"side\":\"TOP\"},\"type\":\"ConnectorPlacement.EquallySpacedRectSide\",\"uuid\":\"fdd70777-e9cf-4317-afb6-cae87f75d5b0\"},{\"content\":{\"connectorIds\":[\"RConn1\"],\"side\":\"BOTTOM\"},\"type\":\"ConnectorPlacement.EquallySpacedRectSide\",\"uuid\":\"2353ed68-b1a1-4775-9ca9-31e268d5443b\"}]},\"type\":\"ConnectorPlacement.EquallySpacedConnector\",\"uuid\":\"d5479f4c-4e65-4791-adcb-73df11f88590\"}],\"packageUris\":[\"http://schema.mathworks.com/mf0/Connector/R2020b\"],\"version\":\"1.0\"}"
  switch_4 : Subsystem
      settings: PortSchema="{\"entries\":[{\"content\":{\"sides\":[{\"content\":{\"connectorIds\":[\"LConn1\"]},\"type\":\"ConnectorPlacement.EquallySpacedRectSide\",\"uuid\":\"9277da8d-d460-43e6-8478-dd662f15d226\"},{\"content\":{\"connectorIds\":[],\"side\":\"RIGHT\"},\"type\":\"ConnectorPlacement.EquallySpacedRectSide\",\"uuid\":\"a7ece396-f1d9-4f4f-a05b-db1fc65d6e1d\"},{\"content\":{\"connectorIds\":[\"LConn2\"],\"side\":\"TOP\"},\"type\":\"ConnectorPlacement.EquallySpacedRectSide\",\"uuid\":\"fdd70777-e9cf-4317-afb6-cae87f75d5b0\"},{\"content\":{\"connectorIds\":[\"RConn1\"],\"side\":\"BOTTOM\"},\"type\":\"ConnectorPlacement.EquallySpacedRectSide\",\"uuid\":\"2353ed68-b1a1-4775-9ca9-31e268d5443b\"}]},\"type\":\"ConnectorPlacement.EquallySpacedConnector\",\"uuid\":\"d5479f4c-4e65-4791-adcb-73df11f88590\"}],\"packageUris\":[\"http://schema.mathworks.com/mf0/Connector/R2020b\"],\"version\":\"1.0\"}"
  uac_out(+) : PMIOPort  Side=Left
  uac_out(-) : PMIOPort  Port=2  Side=Left
  udc(+) : PMIOPort  Port=3  Side=Right
  udc(-) : PMIOPort  Port=4  Side=Right
  wires:
  Bus Selector/4 -> [gate_Q4]  "<gate_cmd_Q2 (signal 4)>"
  Bus Selector/3 -> [gate_Q3]  "<gate_cmd_Q1 (signal 3)>"
  Bus Selector/2 -> [gate_Q2]  "<gate_cmd_Q2 (signal 2)>"
  Bus Selector/1 -> [gate_Q1]  "<gate_cmd_Q1 (signal 1)>"
  gate_commands/1 -> Bus Selector/1
  [gate_Q4] -> Simulink-PS Converter3/1
  [gate_Q3] -> Simulink-PS Converter2/1
  [gate_Q2] -> Simulink-PS Converter1/1
  [gate_Q1] -> Simulink-PS Converter/1
  connections:
  switch_3/RConn1 -- switch_4/LConn2 -- uac_out(-)/RConn1
  switch_1/RConn1 -- switch_2/LConn2 -- uac_out(+)/RConn1
  switch_4/LConn1 -- Simulink-PS Converter3/RConn1
  switch_3/LConn1 -- Simulink-PS Converter2/RConn1
  switch_2/LConn1 -- Simulink-PS Converter1/RConn1
  Simulink-PS Converter/RConn1 -- switch_1/LConn1
  switch_2/RConn1 -- switch_4/RConn1 -- udc(-)/RConn1
  udc(+)/RConn1 -- switch_1/LConn2 -- switch_3/LConn2

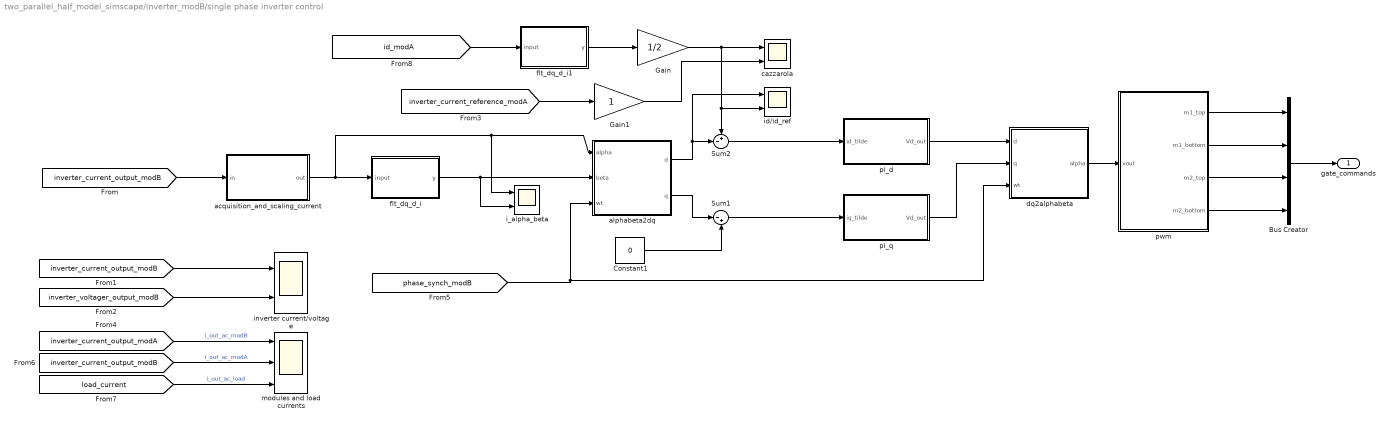
== system two_parallel_half_model_simscape/inverter_modB/single phase inverter control ==
  Bus Creator : BusCreator  Inputs=4
  Constant1 : Constant  Value=0
  Gain : Gain  Gain=1/2
  Gain1 : Gain
  Sum1 : Sum  Inputs=|-+
  Sum2 : Sum  Inputs=+-|
  acquisition_and_scaling_current : Subsystem
  alphabeta2dq : Subsystem
  cazzarola : Scope  NumInputPorts=2
  dq2alphabeta : Subsystem
  flt_dq_d_i : MATLAB Function  TreatAsAtomicUnit=on  SystemSampleTime=ts_inv
  flt_dq_d_i1 : MATLAB Function  TreatAsAtomicUnit=on  SystemSampleTime=ts_inv
  i_alpha_beta : Scope  NumInputPorts=2
  id/id_ref : Scope  NumInputPorts=2
  inverter current/voltage : Scope  NumInputPorts=2
  modules and load currents : Scope  NumInputPorts=3
  pi_d : Subsystem
  pi_q : Subsystem
  pwm : Subsystem
  gate_commands : Outport
  wires:
  [inverter_voltager_output_modB] -> inverter current/voltage/2
  [inverter_current_output_modB] -> inverter current/voltage/1
  [inverter_current_output_modB] -> acquisition_and_scaling_current/1(in)
  acquisition_and_scaling_current/1(out) -> alphabeta2dq/1(alpha), i_alpha_beta/1, flt_dq_d_i/1(input)
  [inverter_current_output_modB] -> modules and load currents/2  "i_out_ac_modA"
  [load_current] -> modules and load currents/3  "i_out_ac_load"
  [inverter_current_output_modA] -> modules and load currents/1  "i_out_ac_modB"
  pwm/4(m2_bottom) -> Bus Creator/4
  pwm/2(m1_bottom) -> Bus Creator/2
  pwm/1(m1_top) -> Bus Creator/1
  Bus Creator/1 -> gate_commands/1
  pwm/3(m2_top) -> Bus Creator/3
  pi_q/1(Vd_out) -> dq2alphabeta/2(q)
  pi_d/1(Vd_out) -> dq2alphabeta/1(d)
  Sum1/1 -> pi_q/1(iq_tilde)
  Sum2/1 -> pi_d/1(id_tilde)
  Constant1/1 -> Sum1/2
  alphabeta2dq/1("d ") -> id/id_ref/1, Sum2/2
  alphabeta2dq/2("q ") -> Sum1/1
  flt_dq_d_i/1(y) -> alphabeta2dq/2(beta), i_alpha_beta/2
  dq2alphabeta/1(alpha) -> pwm/1(vout)
  [phase_synch_modB] -> dq2alphabeta/3(wt), alphabeta2dq/3(wt)
  [id_modA] -> flt_dq_d_i1/1(input)
  flt_dq_d_i1/1(y) -> Gain/1
  Gain/1 -> Sum2/1, id/id_ref/2, cazzarola/1
  [inverter_current_reference_modA] -> Gain1/1
  Gain1/1 -> cazzarola/2

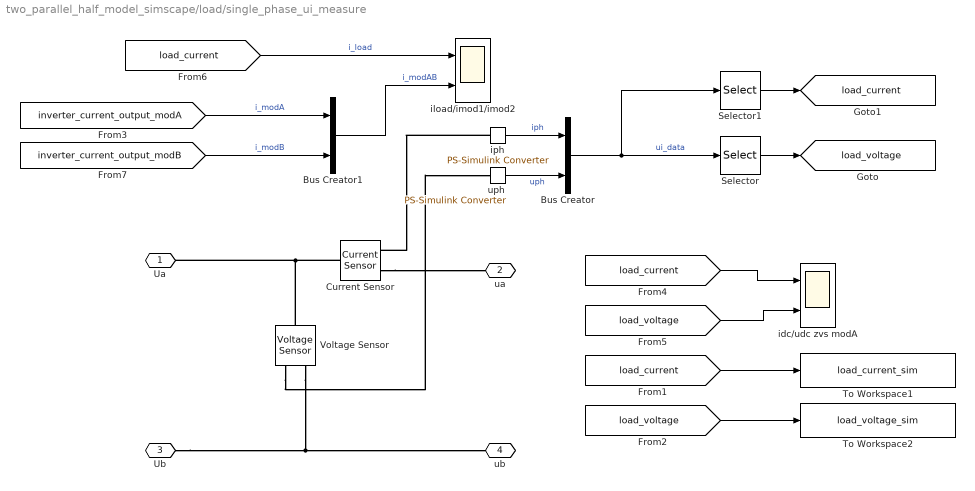
== system two_parallel_half_model_simscape/load/single_phase_ui_measure ==
  Bus Creator : BusCreator  Inputs=2
  Bus Creator1 : BusCreator  Inputs=2
  Current Sensor : fl_lib/Electrical/Electrical Sensors/Current Sensor
  Selector : Selector  InputPortWidth=2  IndexOptions=Index vector (dialog)  Indices=2  OutputSizes=1
  Selector1 : Selector  InputPortWidth=2  IndexOptions=Index vector (dialog)  Indices=1  OutputSizes=1
  To Workspace1 : ToWorkspace  VariableName=load_current_sim  SampleTime=tc
      settings: MaxDataPoints=Nc
  To Workspace2 : ToWorkspace  VariableName=load_voltage_sim  SampleTime=tc
      settings: MaxDataPoints=Nc
  Voltage Sensor : fl_lib/Electrical/Electrical Sensors/Voltage Sensor
  idc/udc zvs modA : Scope  NumInputPorts=2
  iload/imod1/imod2 : Scope  NumInputPorts=2
  iph : nesl_utility/PS-Simulink Converter  PhysicalDomain=network_engine_domain  SubClassName=ps_output  LeftPortType=input  RightPortType=output  PseudoPeriodic=off  Frequencies=[]  VectorFormat=1-D array  Unit=A  AffineConversion=off
  uph : nesl_utility/PS-Simulink Converter  PhysicalDomain=network_engine_domain  SubClassName=ps_output  LeftPortType=input  RightPortType=output  PseudoPeriodic=off  Frequencies=[]  VectorFormat=1-D array  Unit=V  AffineConversion=off
  Ua : PMIOPort  Side=Left
  ua : PMIOPort  Port=2  Side=Right
  Ub : PMIOPort  Port=3  Side=Left
  ub : PMIOPort  Port=4  Side=Right
  tag scope: load_current=global, load_voltage=global
  wires:
  [load_current] -> idc/udc zvs modA/1
  [load_voltage] -> idc/udc zvs modA/2
  Selector1/1 -> [load_current]
  Selector/1 -> [load_voltage]
  Bus Creator/1 -> Selector/1, Selector1/1  "ui_data"
  iph/1 -> Bus Creator/1  "iph"
  uph/1 -> Bus Creator/2  "uph"
  [load_current] -> To Workspace1/1
  [load_voltage] -> To Workspace2/1
  [load_current] -> iload/imod1/imod2/1  "i_load"
  [inverter_current_output_modA] -> Bus Creator1/1  "i_modA"
  [inverter_current_output_modB] -> Bus Creator1/2  "i_modB"
  Bus Creator1/1 -> iload/imod1/imod2/2  "i_modAB"
  connections:
  iph/LConn1 -- Current Sensor/RConn1
  Voltage Sensor/LConn1 -- Current Sensor/LConn1 -- Ua/RConn1
  Current Sensor/RConn2 -- ua/RConn1
  Voltage Sensor/RConn1 -- uph/LConn1
  Voltage Sensor/RConn2 -- Ub/RConn1 -- ub/RConn1

== system two_parallel_half_model_simscape/inverter_modA/single phase inverter/switch_1 ==
  Diode : fl_lib/Electrical/Electrical Elements/Diode  Vf=Vdon_diode V  Ron=Rdon_diode Ohm  Goff=1e-8 1/Ohm  i_specify=off  i_priority=None  i=0 A  i_nominal_specify=off  i_nominal_unit=A  i_nominal_value=1  v_specify=off  v_priority=None  v=0 V  v_nominal_specify=off  v_nominal_unit=V  v_nominal_value=1
  Switch : fl_lib/Electrical/Electrical Elements/Switch  R_closed=Ron Ohm  G_open=1e-8 1/Ohm  Threshold=7.5  i_specify=off  i_priority=None  i=0 A  i_nominal_specify=off  i_nominal_unit=A  i_nominal_value=1  v_specify=off  v_priority=None  v=0 V  v_nominal_specify=off  v_nominal_unit=V  v_nominal_value=1
  G : PMIOPort  Side=Left
  C : PMIOPort  Port=2  Side=Left
  E : PMIOPort  Port=3  Side=Right
  connections:
  Switch/RConn2 -- C/RConn1 -- Diode/RConn1
  Switch/RConn1 -- G/RConn1
  Switch/LConn1 -- E/RConn1 -- Diode/LConn1

== system two_parallel_half_model_simscape/inverter_modA/single phase inverter/switch_2 ==
  Diode : fl_lib/Electrical/Electrical Elements/Diode  Vf=Vdon_diode V  Ron=Rdon_diode Ohm  Goff=1e-8 1/Ohm  i_specify=off  i_priority=None  i=0 A  i_nominal_specify=off  i_nominal_unit=A  i_nominal_value=1  v_specify=off  v_priority=None  v=0 V  v_nominal_specify=off  v_nominal_unit=V  v_nominal_value=1
  Switch : fl_lib/Electrical/Electrical Elements/Switch  R_closed=Ron Ohm  G_open=1e-8 1/Ohm  Threshold=7.5  i_specify=off  i_priority=None  i=0 A  i_nominal_specify=off  i_nominal_unit=A  i_nominal_value=1  v_specify=off  v_priority=None  v=0 V  v_nominal_specify=off  v_nominal_unit=V  v_nominal_value=1
  G : PMIOPort  Side=Left
  C : PMIOPort  Port=2  Side=Left
  E : PMIOPort  Port=3  Side=Right
  connections:
  Diode/LConn1 -- E/RConn1 -- Switch/LConn1
  Switch/RConn1 -- G/RConn1
  Diode/RConn1 -- C/RConn1 -- Switch/RConn2

== system two_parallel_half_model_simscape/inverter_modA/single phase inverter/switch_3 ==
  Diode : fl_lib/Electrical/Electrical Elements/Diode  Vf=Vdon_diode V  Ron=Rdon_diode Ohm  Goff=1e-8 1/Ohm  i_specify=off  i_priority=None  i=0 A  i_nominal_specify=off  i_nominal_unit=A  i_nominal_value=1  v_specify=off  v_priority=None  v=0 V  v_nominal_specify=off  v_nominal_unit=V  v_nominal_value=1
  Switch : fl_lib/Electrical/Electrical Elements/Switch  R_closed=Ron Ohm  G_open=1e-8 1/Ohm  Threshold=7.5  i_specify=off  i_priority=None  i=0 A  i_nominal_specify=off  i_nominal_unit=A  i_nominal_value=1  v_specify=off  v_priority=None  v=0 V  v_nominal_specify=off  v_nominal_unit=V  v_nominal_value=1
  G : PMIOPort  Side=Left
  C : PMIOPort  Port=2  Side=Left
  E : PMIOPort  Port=3  Side=Right
  connections:
  Switch/RConn2 -- C/RConn1 -- Diode/RConn1
  Switch/RConn1 -- G/RConn1
  Switch/LConn1 -- E/RConn1 -- Diode/LConn1

== system two_parallel_half_model_simscape/inverter_modA/single phase inverter/switch_4 ==
  Diode : fl_lib/Electrical/Electrical Elements/Diode  Vf=Vdon_diode V  Ron=Rdon_diode Ohm  Goff=1e-8 1/Ohm  i_specify=off  i_priority=None  i=0 A  i_nominal_specify=off  i_nominal_unit=A  i_nominal_value=1  v_specify=off  v_priority=None  v=0 V  v_nominal_specify=off  v_nominal_unit=V  v_nominal_value=1
  Switch : fl_lib/Electrical/Electrical Elements/Switch  R_closed=Ron Ohm  G_open=1e-8 1/Ohm  Threshold=7.5  i_specify=off  i_priority=None  i=0 A  i_nominal_specify=off  i_nominal_unit=A  i_nominal_value=1  v_specify=off  v_priority=None  v=0 V  v_nominal_specify=off  v_nominal_unit=V  v_nominal_value=1
  G : PMIOPort  Side=Left
  C : PMIOPort  Port=2  Side=Left
  E : PMIOPort  Port=3  Side=Right
  connections:
  Diode/LConn1 -- E/RConn1 -- Switch/LConn1
  Switch/RConn1 -- G/RConn1
  Diode/RConn1 -- C/RConn1 -- Switch/RConn2

== system two_parallel_half_model_simscape/inverter_modA/single phase inverter control/acquisition_and_scaling_current ==
  in : Inport
  1/Ti5 : Gain  Gain=1/I_FS  SaturateOnIntegerOverflow=on  OutDataTypeStr=Inherit: Same as input  ParamDataTypeStr=Inherit: Same as input
  Unit Delay4 : UnitDelay  SampleTime=ts_inv  HasFrameUpgradeWarning=on
  Zero-Order Hold1 : ZeroOrderHold  SampleTime=ts_inv
  out : Outport
  wires:
  in/1 -> Zero-Order Hold1/1
  1/Ti5/1 -> Unit Delay4/1
  Zero-Order Hold1/1 -> 1/Ti5/1
  Unit Delay4/1 -> out/1

== system two_parallel_half_model_simscape/inverter_modA/single phase inverter control/acquisition_and_scaling_voltage ==
  in : Inport
  1/Ti1 : Gain  Gain=1/V_FS  SaturateOnIntegerOverflow=on  OutDataTypeStr=Inherit: Same as input  ParamDataTypeStr=Inherit: Same as input
  Unit Delay4 : UnitDelay  SampleTime=ts_inv  HasFrameUpgradeWarning=on
  Zero-Order Hold2 : ZeroOrderHold  SampleTime=ts_inv
  out : Outport
  wires:
  1/Ti1/1 -> Unit Delay4/1
  Zero-Order Hold2/1 -> 1/Ti1/1
  Unit Delay4/1 -> out/1
  in/1 -> Zero-Order Hold2/1

== system two_parallel_half_model_simscape/inverter_modA/single phase inverter control/alphabeta2dq ==
  note: va=V cos(wt)
      | vb=V cos(wt-2pi/3)
      | vc=V cos(wt+2pi/3)
  alpha : Inport
  beta : Inport  Port=2
  wt : Inport  Port=3
  Product{,1..3} (4 alike) : Product  RndMeth=Zero
  Sum : Sum
  Sum1 : Sum  Inputs=-+
  To Workspace1 : ToWorkspace  VariableName=id_pu_modA_sim  SampleTime=ts_inv
      settings: MaxDataPoints=Ns_inv
  To Workspace2 : ToWorkspace  VariableName=iq_pu_modA_sim  SampleTime=ts_inv
      settings: MaxDataPoints=Ns_inv
  Trigonometric Function : Trigonometry  Operator=cos
  Trigonometric Function1 : Trigonometry
  "d " : Outport  VectorParamsAs1DForOutWhenUnconnected=off
  "q " : Outport  Port=2  VectorParamsAs1DForOutWhenUnconnected=off
  wires:
  wt/1 -> Trigonometric Function1/1, Trigonometric Function/1
  Trigonometric Function/1 -> [cos]
  Trigonometric Function1/1 -> [sin]
  [cos] -> Product/1
  alpha/1 -> Product/2, Product2/2
  Product/1 -> Sum/1
  Product1/1 -> Sum/2
  [sin] -> Product1/1
  beta/1 -> Product1/2, Product3/2
  Sum/1 -> To Workspace1/1, "d "/1
  [sin] -> Product2/1
  Product2/1 -> Sum1/1
  Product3/1 -> Sum1/2
  [cos] -> Product3/1
  Sum1/1 -> To Workspace2/1, "q "/1

== system two_parallel_half_model_simscape/inverter_modA/single phase inverter control/dq2alphabeta ==
  d : Inport
  q : Inport  Port=2
  wt : Inport  Port=3
  Product{,1..3} (4 alike) : Product  RndMeth=Zero
  Sum : Sum  Inputs=+-
  Sum1 : Sum
  Trigonometric Function : Trigonometry  Operator=cos
  Trigonometric Function1 : Trigonometry
  alpha : Outport  VectorParamsAs1DForOutWhenUnconnected=off
  wires:
  [cos] -> Product3/1
  Product3/1 -> Sum1/2
  Product2/1 -> Sum1/1
  [sin] -> Product2/1
  Sum/1 -> alpha/1
  q/1 -> Product3/2, Product1/2
  [sin] -> Product1/1
  Product1/1 -> Sum/2
  Product/1 -> Sum/1
  d/1 -> Product2/2, Product/2
  [cos] -> Product/1
  Trigonometric Function1/1 -> [sin]
  Trigonometric Function/1 -> [cos]
  wt/1 -> Trigonometric Function/1, Trigonometric Function1/1

== system two_parallel_half_model_simscape/inverter_modA/single phase inverter control/pi_d ==
  id_tilde : Inport
  1/Ti : Gain  Gain=kp_i_inv  SaturateOnIntegerOverflow=on  OutDataTypeStr=Inherit: Same as input  ParamDataTypeStr=Inherit: Same as input
  Sum1 : Sum  Inputs=+++  SaturateOnIntegerOverflow=on
  Sum3 : Sum  Inputs=-+  SaturateOnIntegerOverflow=on
  To Workspace3 : ToWorkspace  VariableName=id_ctrl_out_modA_sim  SampleTime=ts_inv
      settings: MaxDataPoints=Ns_inv
  Unit Delay4 : UnitDelay  SampleTime=ts_inv  HasFrameUpgradeWarning=on
  kp2 : Gain  Gain=ki_i_inv*ts_inv  SaturateOnIntegerOverflow=on  OutDataTypeStr=Inherit: Same as input  ParamDataTypeStr=Inherit: Same as input
  ud_out_lim : Saturate  UpperLimit=1  LowerLimit=-1
  "ud_out_lim " : Saturate  UpperLimit=1  LowerLimit=-1
  Vd_out : Outport  VectorParamsAs1DForOutWhenUnconnected=off
  wires:
  id_tilde/1 -> kp2/1, 1/Ti/1
  Sum1/1 -> ud_out_lim/1
  kp2/1 -> Sum1/2
  1/Ti/1 -> Sum1/1, Sum3/1
  Unit Delay4/1 -> Sum1/3
  Sum3/1 -> Unit Delay4/1
  ud_out_lim/1 -> Sum3/2, "ud_out_lim "/1
  "ud_out_lim "/1 -> To Workspace3/1, Vd_out/1

== system two_parallel_half_model_simscape/inverter_modA/single phase inverter control/pi_q ==
  iq_tilde : Inport
  1/Ti : Gain  Gain=kp_i_inv  SaturateOnIntegerOverflow=on  OutDataTypeStr=Inherit: Same as input  ParamDataTypeStr=Inherit: Same as input
  Sum1 : Sum  Inputs=+++  SaturateOnIntegerOverflow=on
  Sum3 : Sum  Inputs=-+  SaturateOnIntegerOverflow=on
  To Workspace3 : ToWorkspace  VariableName=iq_ctrl_out_modA_sim  SampleTime=ts_inv
      settings: MaxDataPoints=Ns_inv
  Unit Delay4 : UnitDelay  SampleTime=ts_inv  HasFrameUpgradeWarning=on
  kp2 : Gain  Gain=ki_i_inv*ts_inv  SaturateOnIntegerOverflow=on  OutDataTypeStr=Inherit: Same as input  ParamDataTypeStr=Inherit: Same as input
  ud_out_lim : Saturate  UpperLimit=1  LowerLimit=-1
  "uq_out_lim " : Saturate  UpperLimit=1  LowerLimit=-1
  Vd_out : Outport  VectorParamsAs1DForOutWhenUnconnected=off
  wires:
  "uq_out_lim "/1 -> Vd_out/1, To Workspace3/1
  ud_out_lim/1 -> "uq_out_lim "/1, Sum3/2
  Sum3/1 -> Unit Delay4/1
  Unit Delay4/1 -> Sum1/3
  1/Ti/1 -> Sum3/1, Sum1/1
  kp2/1 -> Sum1/2
  Sum1/1 -> ud_out_lim/1
  iq_tilde/1 -> 1/Ti/1, kp2/1

== system two_parallel_half_model_simscape/inverter_modA/single phase inverter control/pi_v ==
  e : Inport
  1/Ti : Gain  Gain=kp_v_inv  SaturateOnIntegerOverflow=on  OutDataTypeStr=Inherit: Same as input  ParamDataTypeStr=Inherit: Same as input
  Sum1 : Sum  Inputs=+++  SaturateOnIntegerOverflow=on
  Sum3 : Sum  Inputs=-+  SaturateOnIntegerOverflow=on
  To Workspace3 : ToWorkspace  VariableName=v_ctrl_out_modA_sim  SampleTime=ts_inv
      settings: MaxDataPoints=Ns_inv
  Unit Delay4 : UnitDelay  SampleTime=ts_inv  HasFrameUpgradeWarning=on
  i_out_lim : Saturate  UpperLimit=0.869565217391304  LowerLimit=0
  kp2 : Gain  Gain=ki_v_inv*ts_inv  SaturateOnIntegerOverflow=on  OutDataTypeStr=Inherit: Same as input  ParamDataTypeStr=Inherit: Same as input
  i_ref_internal : Outport  VectorParamsAs1DForOutWhenUnconnected=off
  wires:
  i_out_lim/1 -> i_ref_internal/1, To Workspace3/1, Sum3/2
  Sum3/1 -> Unit Delay4/1
  Unit Delay4/1 -> Sum1/3
  1/Ti/1 -> Sum3/1, Sum1/1
  kp2/1 -> Sum1/2
  Sum1/1 -> i_out_lim/1
  e/1 -> kp2/1, 1/Ti/1

== system two_parallel_half_model_simscape/inverter_modA/single phase inverter control/pwm ==
  vout : Inport
  Constant : Constant  Value=0
  Constant1 : Constant
  Constant2 : Constant
  Constant3 : Constant
  Gain1 : Gain  Gain=1/2
  Gain2 : Gain
  Gain3 : Gain  Gain=1/2
  Gain4 : Gain  Gain=-1
  PWM generator 1 : Subsystem  mask{f=fPWM_INV, m_up=1, m_low=0, dead_time=0, pos_cmd_gate=15, neg_cmd_gate=-10, polarity=-1}
      mask prompts: f "Frequency (Hz)"; m_up "Max Input Modulation Value"; m_low "Min Input Modulation Value"; dead_time "Dead Time (s)"; pos_cmd_gate "Positive Gate Voltage (V)"; neg_cmd_gate "Negative Gate Voltage (V)"; polarity "Polarity (pu)"
  PWM generator 2 : Subsystem  mask{f=fPWM_INV, m_up=1, m_low=0, dead_time=0, pos_cmd_gate=15, neg_cmd_gate=-10, polarity=-1}
      mask prompts: f "Frequency (Hz)"; m_up "Max Input Modulation Value"; m_low "Min Input Modulation Value"; dead_time "Dead Time (s)"; pos_cmd_gate "Positive Gate Voltage (V)"; neg_cmd_gate "Negative Gate Voltage (V)"; polarity "Polarity (pu)"
  Sum : Sum  Inputs=|++
  Sum1 : Sum  Inputs=|++
  m1_top : Outport
  m1_bottom : Outport  Port=2
  m2_top : Outport  Port=3
  m2_bottom : Outport  Port=4
  wires:
  PWM generator 1/1(m1) -> m1_top/1  "gate_cmd_Q1"
  PWM generator 1/2(m2) -> m1_bottom/1  "gate_cmd_Q2"
  PWM generator 2/2(m2) -> m2_bottom/1  "gate_cmd_Q2"
  PWM generator 2/1(m1) -> m2_top/1  "gate_cmd_Q1"
  Constant/1 -> PWM generator 2/2(phase), PWM generator 1/2(phase)
  Constant1/1 -> PWM generator 2/3(polarity_input), PWM generator 1/3(polarity_input)
  Gain2/1 -> Sum/1
  Sum/1 -> Gain1/1
  Constant2/1 -> Sum/2
  Gain1/1 -> PWM generator 1/1(m_index)
  Constant3/1 -> Sum1/2
  Sum1/1 -> Gain3/1
  Gain4/1 -> Sum1/1
  Gain3/1 -> PWM generator 2/1(m_index)
  vout/1 -> Gain4/1, Gain2/1
